simulink model "Hil_Climbers_Integrated_V5"  (R2021a)
settings: Solver=VariableStepAuto  StartTime=0.0  StopTime=10.0  RelTol=1e-3
settings Model: Creator=Sai229  LastModifiedBy=achu

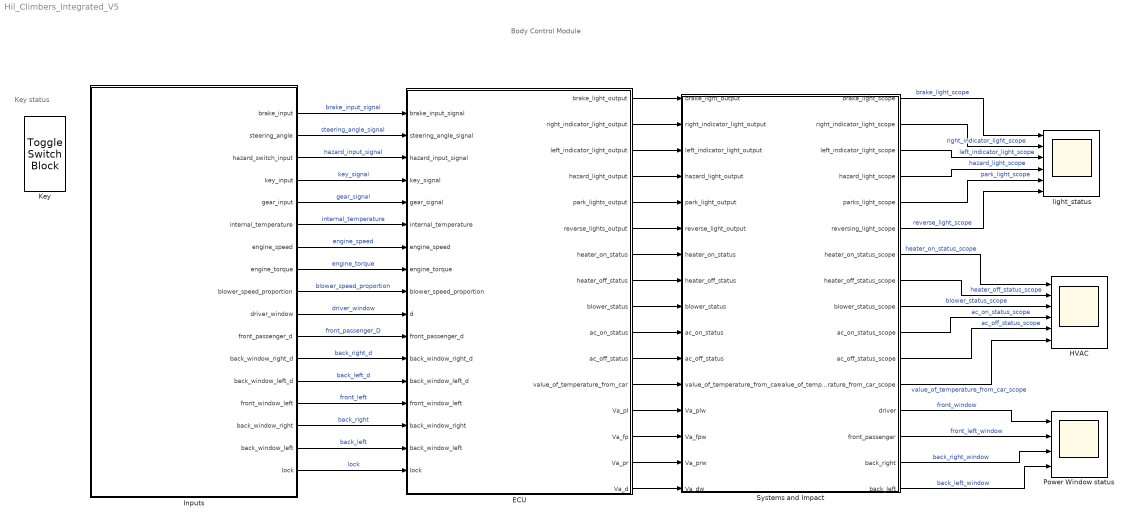
== system Hil_Climbers_Integrated_V5 ==
  note: Key status
  note: Body Control Module
  " ECU" : Subsystem
  HVAC : Scope  NumInputPorts=6
  Inputs : Subsystem
  Key : ToggleSwitchBlock  LabelPosition=Hide
      settings: Values={{'Off', 'On'}, [0 1]}
  Power Window status : Scope  NumInputPorts=4
  Systems and Impact : Subsystem
  light_status : Scope  NumInputPorts=6
  wires:
  Systems and Impact/1(brake_light_scope) -> light_status/1  "brake_light_scope"
  Systems and Impact/5(parks_light_scope) -> light_status/5  "park_light_scope"
  Systems and Impact/4(hazard_light_scope) -> light_status/4  "hazard_light_scope"
  Systems and Impact/6(reversing_light_scope) -> light_status/6  "reverse_light_scope"
  Systems and Impact/3(left_indicator_light_scope) -> light_status/3  "left_indicator_light_scope"
  Systems and Impact/2(right_indicator_light_scope) -> light_status/2  "right_indicator_light_scope"
  Inputs/1(brake_input) -> " ECU"/1(brake_input_signal)  "brake_input_signal"
  Inputs/2(steering_angle) -> " ECU"/2(steering_angle_signal)  "steering_angle_signal"
  Inputs/3(hazard_switch_input) -> " ECU"/3(hazard_input_signal)  "hazard_input_signal"
  Inputs/4(key_input) -> " ECU"/4(key_signal)  "key_signal"
  Inputs/5(gear_input) -> " ECU"/5(gear_signal)  "gear_signal"
  Inputs/6(internal_temperature) -> " ECU"/6(internal_temperature)  "internal_temperature"
  Inputs/9(blower_speed_proportion) -> " ECU"/9(blower_speed_proportion)  "blower_speed_proportion"
  Inputs/10(driver_window) -> " ECU"/10(d)  "driver_window"
  Inputs/11(front_passenger_d) -> " ECU"/11(front_passenger_d)  "front_passenger_D"
  Inputs/12(back_window_right_d) -> " ECU"/12(back_window_right_d)  "back_right_d"
  Inputs/13(back_window_left_d) -> " ECU"/13(back_window_left_d)  "back_left_d"
  Inputs/14(front_window_left) -> " ECU"/14(front_window_left)  "front_left"
  Inputs/15(back_window_right) -> " ECU"/15(back_window_right)  "back_right"
  Inputs/16(back_window_left) -> " ECU"/16(back_window_left)  "back_left"
  " ECU"/1(brake_light_output) -> Systems and Impact/1(brake_light_output)
  " ECU"/2(right_indicator_light_output) -> Systems and Impact/2(right_indicator_light_output)
  " ECU"/3(left_indicator_light_output) -> Systems and Impact/3(left_indicator_light_output)
  " ECU"/4(hazard_light_output) -> Systems and Impact/4(hazard_light_output)
  " ECU"/5(park_lights_output) -> Systems and Impact/5(park_light_output)
  " ECU"/6(reverse_lights_output) -> Systems and Impact/6(reverse_light_output)
  " ECU"/7(heater_on_status) -> Systems and Impact/7(heater_on_status)
  " ECU"/8(heater_off_status) -> Systems and Impact/8(heater_off_status)
  " ECU"/9(blower_status) -> Systems and Impact/9(blower_status)
  " ECU"/10(ac_on_status) -> Systems and Impact/10(ac_on_status)
  " ECU"/11(ac_off_status) -> Systems and Impact/11(ac_off_status)
  " ECU"/12(value_of_temperature_from_car) -> Systems and Impact/12(value_of_temperature_from_car)
  " ECU"/13(Va_pl) -> Systems and Impact/13(Va_plw)
  " ECU"/14(Va_fp) -> Systems and Impact/14(Va_fpw)
  " ECU"/15(Va_pr) -> Systems and Impact/15(Va_prw)
  " ECU"/16(Va_d) -> Systems and Impact/16(Va_dw)
  Systems and Impact/13(driver) -> Power Window status/1  "front_window"
  Systems and Impact/14(front_passenger) -> Power Window status/2  "front_left_window"
  Systems and Impact/15(back_right) -> Power Window status/3  "back_right_window"
  Systems and Impact/16(back_left) -> Power Window status/4  "back_left_window"
  Inputs/17(lock) -> " ECU"/17(lock)  "lock"
  Systems and Impact/7(heater_on_status_scope) -> HVAC/1  "heater_on_status_scope"
  Systems and Impact/8(heater_off_status_scope) -> HVAC/2  "heater_off_status_scope"
  Systems and Impact/9(blower_status_scope) -> HVAC/3  "blower_status_scope"
  Systems and Impact/10(ac_on_status_scope) -> HVAC/4  "ac_on_status_scope"
  Systems and Impact/11(ac_off_status_scope) -> HVAC/5  "ac_off_status_scope"
  Systems and Impact/12(value_of_temperature_from_car_scope) -> HVAC/6  "value_of_temperature_from_car_scope"
  Inputs/8(engine_torque) -> " ECU"/8(engine_torque)  "engine_torque"
  Inputs/7(engine_speed) -> " ECU"/7(engine_speed)  "engine_speed"

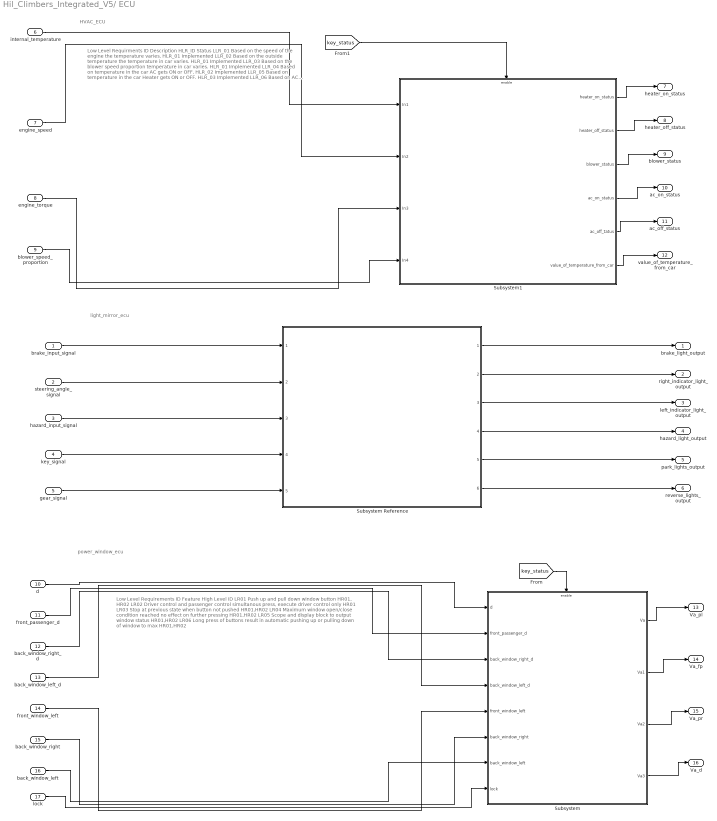
== system Hil_Climbers_Integrated_V5/ ECU ==
  note: light_mirror_ecu
  note: power_window_ecu
  note: HVAC_ECU
  note: Low Level Requirments
      | ID
      | Description
      | HLR_ID
      | Status
      |
      | LLR_01
      | Based on the speed of the engine the temperature varies.
      | HLR_01
      | Implemented
      |
      | LLR_02
      | Based on the outside temperature the temperature in car varies.
      | HLR_01
      | Implemented
      |
      | LLR_03
      | Based on the blower speed proportion temperature in car varies.
      | HLR_01
      | Implemented
      |
      | LLR_04
      | Based on temperature in the car AC gets ON or OFF.
      | HLR_02
      | Implemented
      |
      | LLR_05
      | Based on temperature in the car Heater gets ON or OFF.
      | HLR_03
      | Implemented
      |
      | LLR_06
      | Based on AC status Blower works.
      | HLR_04
      | Implemented
      |
      | LOGIC:
      | STEP 1. Taking values of engine temperature and comp Torque and multipled and given to efficiency(gain).
      | STEP 2. Blower speed proportion and given toMaximum flow rate(gain).
      | STEP 3. Both values were given to divide block.
      | STEP 4. Internal Temperature is in degrees and after it converted into kelvin.
      | STEP 5. Subtract of both values, then the temperature will display on the Display block.
      | 1.Based on temperature the AC is getting on.
      | a.If the value(temperature) is greater than 23 then AC should be on.
      | b.Else the AC should be off.
      | 2. Based on AC status Blower Works.
      | 3. Based on temperature the Blower is getting on.
      | a.If the value(temperature) is less than 18 then Heater should be on.
      | b.Else the Heater should be off.
  note: Low Level Requirements
      |
      | ID
      | Feature
      | High Level ID
      |
      | LR01
      | Push up and pull down window button
      | HR01, HR02
      |
      | LR02
      | Driver control and passenger control simultanous press, execute driver control only
      | HR01
      |
      | LR03
      | Stop at previous state when button not pushed
      | HR01,HR02
      |
      | LR04
      | Maximum window open/close condition reached no effect on further pressing
      | HR01,HR02
      |
      | LR05
      | Scope and display block to output window status
      | HR01,HR02
      |
      | LR06
      | Long press of buttons result in automatic pushing up or pulling down of window to max
      | HR01,HR02
  brake_input_signal : Inport
  steering_angle_signal : Inport  Port=2
  hazard_input_signal : Inport  Port=3
  key_signal : Inport  Port=4
  gear_signal : Inport  Port=5
  internal_temperature : Inport  Port=6
  engine_speed : Inport  Port=7
  engine_torque : Inport  Port=8
  blower_speed_proportion : Inport  Port=9
  d : Inport  Port=10
  front_passenger_d : Inport  Port=11
  back_window_right_d : Inport  Port=12
  back_window_left_d : Inport  Port=13
  front_window_left : Inport  Port=14
  back_window_right : Inport  Port=15
  back_window_left : Inport  Port=16
  lock : Inport  Port=17
  Subsystem : Subsystem
  Subsystem Reference : Subsystem  ReferencedSubsystem=LRLM_ECU
  Subsystem1 : Subsystem
  brake_light_output : Outport
  right_indicator_light_output : Outport  Port=2
  left_indicator_light_output : Outport  Port=3
  hazard_light_output : Outport  Port=4
  park_lights_output : Outport  Port=5
  reverse_lights_output : Outport  Port=6
  heater_on_status : Outport  Port=7
  heater_off_status : Outport  Port=8
  blower_status : Outport  Port=9
  ac_on_status : Outport  Port=10
  ac_off_status : Outport  Port=11
  value_of_temperature_from_car : Outport  Port=12
  Va_pl : Outport  Port=13
  Va_fp : Outport  Port=14
  Va_pr : Outport  Port=15
  Va_d : Outport  Port=16
  wires:
  Subsystem1/1(heater_on_status) -> heater_on_status/1
  Subsystem1/2(heater_off_status) -> heater_off_status/1
  Subsystem1/3(blower_status) -> blower_status/1
  Subsystem1/4(ac_on_status) -> ac_on_status/1
  Subsystem1/5(ac_off_tatus) -> ac_off_status/1
  Subsystem1/6(value_of_temperature_from_car) -> value_of_temperature_from_car/1
  [key_status] -> Subsystem1/Enable
  blower_speed_proportion/1 -> Subsystem1/4(In4)
  engine_speed/1 -> Subsystem1/2(In2)
  internal_temperature/1 -> Subsystem1/1(In1)
  engine_torque/1 -> Subsystem1/3(In3)
  Subsystem/1(Va) -> Va_pl/1
  Subsystem/2(Va1) -> Va_fp/1
  Subsystem/3(Va2) -> Va_pr/1
  Subsystem/4(Va3) -> Va_d/1
  back_window_left_d/1 -> Subsystem/4(back_window_left_d)
  [key_status] -> Subsystem/Enable
  front_window_left/1 -> Subsystem/5(front_window_left)
  front_passenger_d/1 -> Subsystem/2(front_passenger_d)
  back_window_left/1 -> Subsystem/7(back_window_left)
  back_window_right_d/1 -> Subsystem/3(back_window_right_d)
  lock/1 -> Subsystem/8(lock)
  back_window_right/1 -> Subsystem/6(back_window_right)
  d/1 -> Subsystem/1(d)
  Subsystem Reference/1 -> brake_light_output/1
  Subsystem Reference/2 -> right_indicator_light_output/1
  Subsystem Reference/3 -> left_indicator_light_output/1
  Subsystem Reference/4 -> hazard_light_output/1
  Subsystem Reference/5 -> park_lights_output/1
  Subsystem Reference/6 -> reverse_lights_output/1
  hazard_input_signal/1 -> Subsystem Reference/3
  brake_input_signal/1 -> Subsystem Reference/1
  key_signal/1 -> Subsystem Reference/4
  gear_signal/1 -> Subsystem Reference/5
  steering_angle_signal/1 -> Subsystem Reference/2

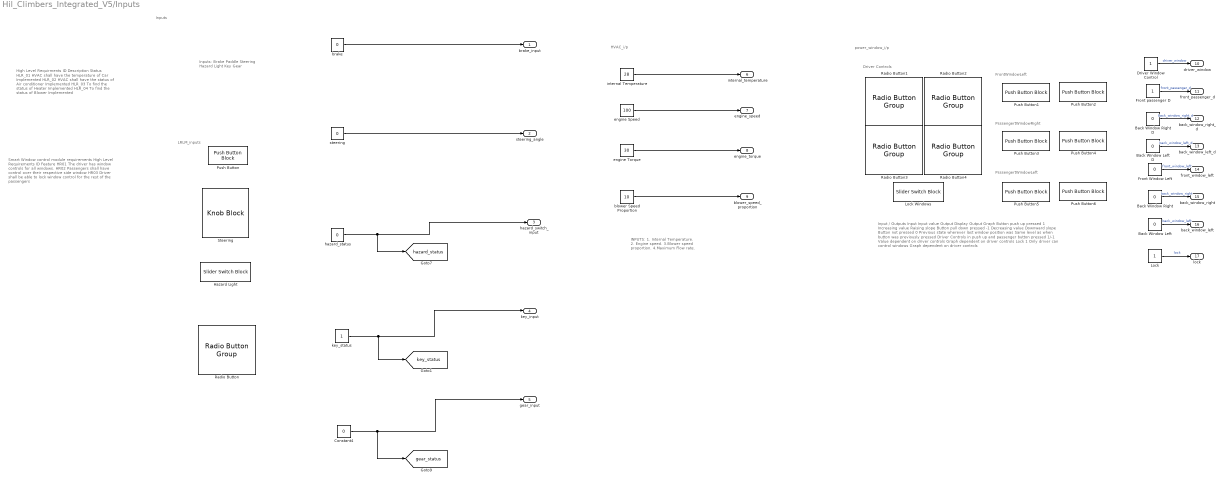
== system Hil_Climbers_Integrated_V5/Inputs ==
  note: HVAC_i/p
  note: power_window_i/p
  note: Inputs
  note: LRLM_inputs
  note: Inputs:
      | Brake Paddle
      | Steering
      | Hazard Light
      | Key
      | Gear
  note: Input / Outputs
      |
      | Input
      | Input value
      | Output Display
      | Output Graph
      |
      | Button push up pressed
      | 1
      | Increasing value
      | Raising slope
      |
      | Button pull down pressed
      | -1
      | Decreasing value
      | Downward slope
      |
      | Button not pressed
      | 0
      | Previous state wherever last window position was
      | Same level as when button was previously pressed
      |
      | Driver Controls in push up and passenger button pressed
      | 1/-1
      | Value dependent on driver controls
      | Graph dependent on driver controls
      |
      | Lock
      | 1
      | Only driver can control windows
      | Graph dependent on driver controls
  note: PsssengertWindowRight
  note: Driver Controls
  note: FrontWindowLeft
  note: PsssengertWindowLeft
  note: INPUTS:
      | 1. Internal Temperature.
      | 2. Engine speed.
      | 3.Blower speed proportion.
      | 4.Maximum Flow rate.
  note: High Level Requirments
      |
      | ID
      | Description
      | Status
      |
      | HLR_01
      | HVAC shall have the temperature of Car
      | Implemented
      |
      | HLR_02
      | HVAC shall have the status of Air conditioner
      | Implemented
      |
      | HLR_03
      | To find the status of Heater
      | Implemented
      |
      | HLR_04
      | To find the status of Blower
      | Implemented
  note: Smart Window control module requirements
      |
      | High Level Requirements
      |
      | ID
      | Feature
      |
      | HR01
      | The driver has window controls for all windows.
      |
      | HR02
      | Passengers shall have control over their respective side window
      |
      | HR03
      | Driver shall be able to lock window control for the rest of the passengers
  Back Window Left : Constant  Value=0
  Back Window Left D : Constant  Value=0
  Back Window Right : Constant  Value=0
  Back Window Right D : Constant  Value=0
  Constant4 : Constant  Value=0
  Driver Window Control : Constant
  Front Window Left : Constant  Value=0
  Front passenger D : Constant
  Hazard Light : SliderSwitchBlock  LabelPosition=Hide
      settings: Values={{'Off', 'On'}, [0 1]}
  Lock : Constant
  Lock Windows : SliderSwitchBlock
      settings: Values={{'Unlock', 'Lock'}, [0 1]}
  Push Button : PushButtonBlock  ButtonText=Brake
  Push Button1 : PushButtonBlock  ButtonText=Push up window
  Push Button2 : PushButtonBlock  ButtonText=Pull down window  OnValue=-1
  Push Button3 : PushButtonBlock  ButtonText=Push up window
  Push Button4 : PushButtonBlock  ButtonText=Pull down window  OnValue=-1
  Push Button5 : PushButtonBlock  ButtonText=Push up window
  Push Button6 : PushButtonBlock  ButtonText=Pull down window  OnValue=-1
  Radio Button : RadioButtonGroup  LabelPosition=Hide  SelectedLabel=Neutral  ButtonGroupName=Gear
      settings: Values={{'Neutral', 'Drive', 'Park', 'Reverse'}, [0 1 2 3]}
  Radio Button1 : RadioButtonGroup  LabelPosition=Hide  SelectedLabel=Stop  ButtonGroupName=Driver Window Controls
      settings: Values={{'Open', 'Stop', 'Close'}, [1 0 -1]}
  Radio Button2 : RadioButtonGroup  LabelPosition=Hide  SelectedLabel=Stop  ButtonGroupName=Front Passenger
      settings: Values={{'Open', 'Stop', 'Close'}, [1 0 -1]}
  Radio Button3 : RadioButtonGroup  LabelPosition=Hide  SelectedLabel=Stop  ButtonGroupName=Back Window Right
      settings: Values={{'Open', 'Stop', 'Close'}, [1 0 -1]}
  Radio Button4 : RadioButtonGroup  LabelPosition=Hide  SelectedLabel=Stop  ButtonGroupName=Back Window Left
      settings: Values={{'Open', 'Stop', 'Close'}, [1 0 -1]}
  Steering : KnobBlock  LabelPosition=Hide  ScaleMin=-50  ScaleMax=50  TickInterval=10
  blower Speed Proportion : Constant  Value=10
  brake : Constant  Value=0
  engine Speed : Constant  Value=100
  engine Torque : Constant  Value=30
  hazard_status : Constant  Value=0
  internal Temperature : Constant  Value=28
  key_status : Constant
  steering : Constant  Value=0
  brake_input : Outport
  steering_angle : Outport  Port=2
  hazard_switch_input : Outport  Port=3
  key_input : Outport  Port=4
  gear_input : Outport  Port=5
  internal_temperature : Outport  Port=6
  engine_speed : Outport  Port=7
  engine_torque : Outport  Port=8
  blower_speed_proportion : Outport  Port=9
  driver_window : Outport  Port=10
  front_passenger_d : Outport  Port=11
  back_window_right_d : Outport  Port=12
  back_window_left_d : Outport  Port=13
  front_window_left : Outport  Port=14
  back_window_right : Outport  Port=15
  back_window_left : Outport  Port=16
  lock : Outport  Port=17
  tag scope: gear_status=global, hazard_status=global, key_status=global
  wires:
  brake/1 -> brake_input/1
  Constant4/1 -> [gear_status], gear_input/1
  steering/1 -> steering_angle/1
  key_status/1 -> [key_status], key_input/1
  hazard_status/1 -> [hazard_status], hazard_switch_input/1
  Front passenger D/1 -> front_passenger_d/1  "front_passenger_d"
  Back Window Left D/1 -> back_window_left_d/1  "back_window_left_d"
  Driver Window Control/1 -> driver_window/1  "driver_window"
  Back Window Right/1 -> back_window_right/1  "back_window_right"
  Front Window Left/1 -> front_window_left/1  "front_window_left"
  Back Window Left/1 -> back_window_left/1  "back_window_left"
  Back Window Right D/1 -> back_window_right_d/1  "back_window_right_d"
  Lock/1 -> lock/1  "lock"
  internal Temperature/1 -> internal_temperature/1
  engine Speed/1 -> engine_speed/1
  engine Torque/1 -> engine_torque/1
  blower Speed Proportion/1 -> blower_speed_proportion/1

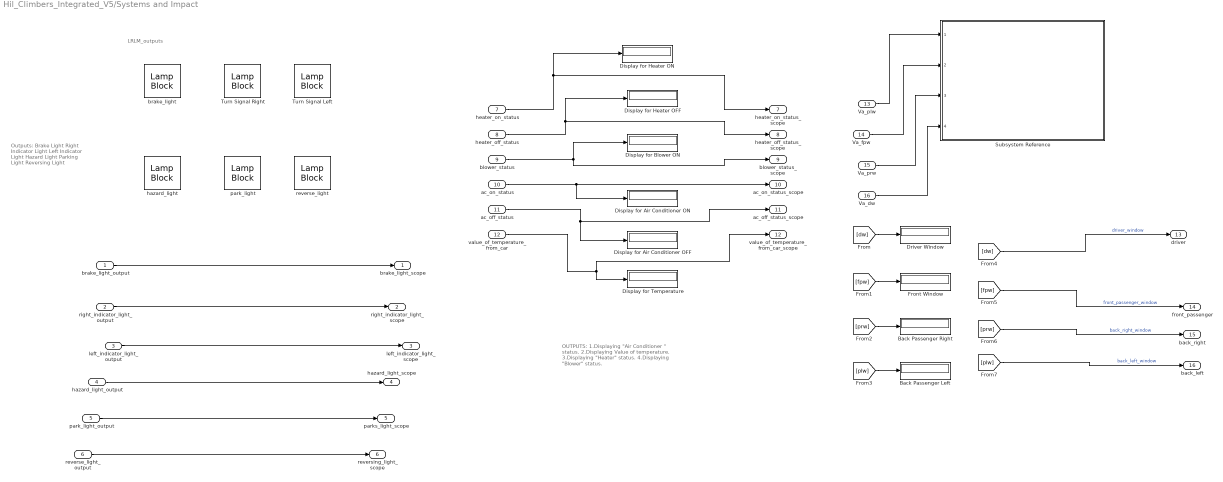
== system Hil_Climbers_Integrated_V5/Systems and Impact ==
  note: OUTPUTS:
      | 1.Displaying "Air Conditioner " status.
      | 2.Displaying Value of temperature.
      | 3.Displaying "Heater" status.
      | 4.Displaying "Blower" status.
  note: Outputs:
      | Brake Light
      | Right Indicator Light
      | Left Indicator Light
      | Hazard Light
      | Parking Light
      | Reversing Light
  note: LRLM_outputs
  brake_light_output : Inport
  right_indicator_light_output : Inport  Port=2
  left_indicator_light_output : Inport  Port=3
  hazard_light_output : Inport  Port=4
  park_light_output : Inport  Port=5
  reverse_light_output : Inport  Port=6
  heater_on_status : Inport  Port=7
  heater_off_status : Inport  Port=8
  blower_status : Inport  Port=9
  ac_on_status : Inport  Port=10
  ac_off_status : Inport  Port=11
  value_of_temperature_from_car : Inport  Port=12
  Va_plw : Inport  Port=13
  Va_fpw : Inport  Port=14
  Va_prw : Inport  Port=15
  Va_dw : Inport  Port=16
  Back Passenger Left : Display
  Back Passenger Right : Display
  Display for Air Conditioner OFF : Display
  Display for Air Conditioner ON : Display
  Display for Blower ON : Display
  Display for Heater OFF : Display
  Display for Heater ON : Display
  Display for Temperature : Display
  Driver Window : Display
  Front Window : Display
  Subsystem Reference : Subsystem  ReferencedSubsystem=power_window_system_impact
  Turn Signal Left : LampBlock  LabelPosition=Hide  Icon=TurnSignalLeft
  Turn Signal Right : LampBlock  LabelPosition=Hide  Icon=TurnSignalRight
  brake_light : LampBlock  LabelPosition=Hide  Icon=LightingSwitch
  hazard_light : LampBlock  LabelPosition=Hide  Icon=Hazards
  park_light : LampBlock  Icon=ParkingAssistance
  reverse_light : LampBlock  Icon=RearFogLight
  brake_light_scope : Outport
  right_indicator_light_scope : Outport  Port=2
  left_indicator_light_scope : Outport  Port=3
  hazard_light_scope : Outport  Port=4
  parks_light_scope : Outport  Port=5
  reversing_light_scope : Outport  Port=6
  heater_on_status_scope : Outport  Port=7
  heater_off_status_scope : Outport  Port=8
  blower_status_scope : Outport  Port=9
  ac_on_status_scope : Outport  Port=10
  ac_off_status_scope : Outport  Port=11
  value_of_temperature_from_car_scope : Outport  Port=12
  driver : Outport  Port=13
  front_passenger : Outport  Port=14
  back_right : Outport  Port=15
  back_left : Outport  Port=16
  wires:
  hazard_light_output/1 -> hazard_light_scope/1
  reverse_light_output/1 -> reversing_light_scope/1
  park_light_output/1 -> parks_light_scope/1
  left_indicator_light_output/1 -> left_indicator_light_scope/1
  right_indicator_light_output/1 -> right_indicator_light_scope/1
  brake_light_output/1 -> brake_light_scope/1
  heater_off_status/1 -> heater_off_status_scope/1, Display for Heater OFF/1
  ac_on_status/1 -> ac_on_status_scope/1, Display for Air Conditioner ON/1
  blower_status/1 -> blower_status_scope/1, Display for Blower ON/1
  ac_off_status/1 -> ac_off_status_scope/1, Display for Air Conditioner OFF/1
  heater_on_status/1 -> heater_on_status_scope/1, Display for Heater ON/1
  value_of_temperature_from_car/1 -> value_of_temperature_from_car_scope/1, Display for Temperature/1
  Va_plw/1 -> Subsystem Reference/1
  Va_fpw/1 -> Subsystem Reference/2
  Va_prw/1 -> Subsystem Reference/3
  Va_dw/1 -> Subsystem Reference/4
  [plw] -> Back Passenger Left/1
  [prw] -> Back Passenger Right/1
  [fpw] -> Front Window/1
  [dw] -> driver/1  "driver_window"
  [fpw] -> front_passenger/1  "front_passenger_window"
  [dw] -> Driver Window/1
  [prw] -> back_right/1  "back_right_window"
  [plw] -> back_left/1  "back_left_window"

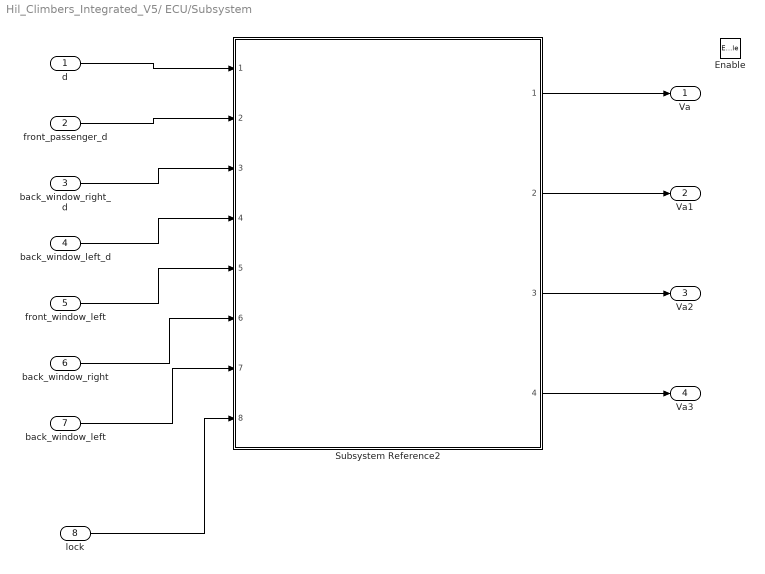
== system Hil_Climbers_Integrated_V5/ ECU/Subsystem ==
  d : Inport
  front_passenger_d : Inport  Port=2
  back_window_right_d : Inport  Port=3
  back_window_left_d : Inport  Port=4
  front_window_left : Inport  Port=5
  back_window_right : Inport  Port=6
  back_window_left : Inport  Port=7
  lock : Inport  Port=8
  Enable : EnablePort  StatesWhenEnabling=reset
  Subsystem Reference2 : Subsystem  ReferencedSubsystem=power_window_ECU
  Va : Outport
  Va1 : Outport  Port=2
  Va2 : Outport  Port=3
  Va3 : Outport  Port=4
  wires:
  Subsystem Reference2/3 -> Va2/1
  Subsystem Reference2/1 -> Va/1
  Subsystem Reference2/2 -> Va1/1
  front_passenger_d/1 -> Subsystem Reference2/2
  back_window_left/1 -> Subsystem Reference2/7
  back_window_right_d/1 -> Subsystem Reference2/3
  back_window_left_d/1 -> Subsystem Reference2/4
  back_window_right/1 -> Subsystem Reference2/6
  Subsystem Reference2/4 -> Va3/1
  front_window_left/1 -> Subsystem Reference2/5
  d/1 -> Subsystem Reference2/1
  lock/1 -> Subsystem Reference2/8

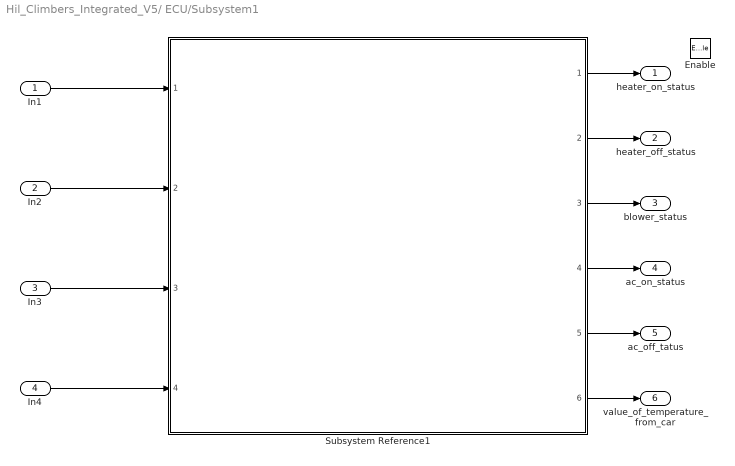
== system Hil_Climbers_Integrated_V5/ ECU/Subsystem1 ==
  In1 : Inport
  In2 : Inport  Port=2
  In3 : Inport  Port=3
  In4 : Inport  Port=4
  Enable : EnablePort  StatesWhenEnabling=reset
  Subsystem Reference1 : Subsystem  ReferencedSubsystem=HVAC_ECU
  heater_on_status : Outport
  heater_off_status : Outport  Port=2
  blower_status : Outport  Port=3
  ac_on_status : Outport  Port=4
  ac_off_tatus : Outport  Port=5
  value_of_temperature_from_car : Outport  Port=6
  wires:
  Subsystem Reference1/2 -> heater_off_status/1
  In2/1 -> Subsystem Reference1/2
  In1/1 -> Subsystem Reference1/1
  Subsystem Reference1/6 -> value_of_temperature_from_car/1
  Subsystem Reference1/5 -> ac_off_tatus/1
  Subsystem Reference1/1 -> heater_on_status/1
  Subsystem Reference1/3 -> blower_status/1
  In3/1 -> Subsystem Reference1/3
  Subsystem Reference1/4 -> ac_on_status/1
  In4/1 -> Subsystem Reference1/4
